simulink model "AirManifold"  (R2019a)
settings: Solver=ode15s  StartTime=0.0  StopTime=5000  RelTol=1e-3
libraries: fl_lib x15, nesl_utility x4, SimscapeFluids_lib x2
(part 2 of 2)

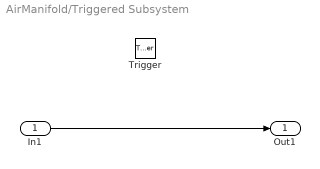
== system AirManifold/Triggered Subsystem ==
  In1 : Inport
  Trigger : TriggerPort  TriggerType=falling  VariantControl=Variant
  Out1 : Outport
  wires:
  In1/1 -> Out1/1

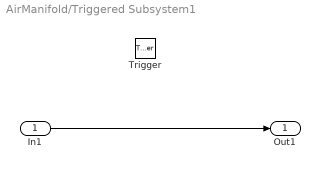
== system AirManifold/Triggered Subsystem1 ==
  In1 : Inport
  Trigger : TriggerPort  VariantControl=Variant
  Out1 : Outport
  wires:
  In1/1 -> Out1/1
